simulink library "UDP_bus_create_lib"  (Simulink 7.2)
settings: Solver=ode45  StartTime=0.0  StopTime=10.0  RelTol=1e-3
libraries: simulink x1, UDP_lib x1
settings Model: Creator=cbuttril  LastModifiedBy=gtmdev

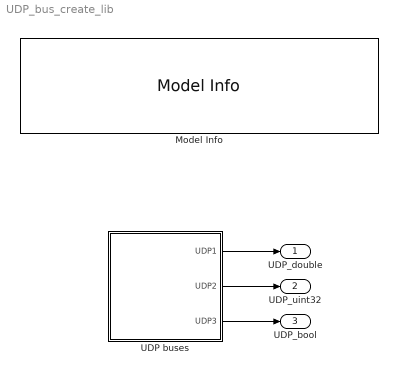
== system UDP_bus_create_lib ==
  Model Info : simulink/Model-Wide Utilities/Model Info  SystemSampleTime=-1  InitialBlockCM=None  BlockCM=None  Frame=on  DisplayStringWithTags=|  HorizontalTextAlignment=Center  LeftAlignmentValue=0.5  SourceBlockDiagram=UDP_bus_create_lib  TagMaxNumber=20
      | Developed using Matlab Release 2008b
      | 
      | SVN:%<ModelVersion>
      | Last modifed by %<LastModifiedBy> on %<LastModificationDate>
  UDP buses : Subsystem
  UDP_double : Outport  OutDataType=sfix(16)  OutScaling=2^0
  UDP_uint32 : Outport  Port=2  OutDataType=sfix(16)  OutScaling=2^0
  UDP_bool : Outport  Port=3  OutDataType=sfix(16)  OutScaling=2^0
  wires:
  UDP buses/1(UDP1) -> UDP_double/1
  UDP buses/2(UDP2) -> UDP_uint32/1
  UDP buses/3(UDP3) -> UDP_bool/1

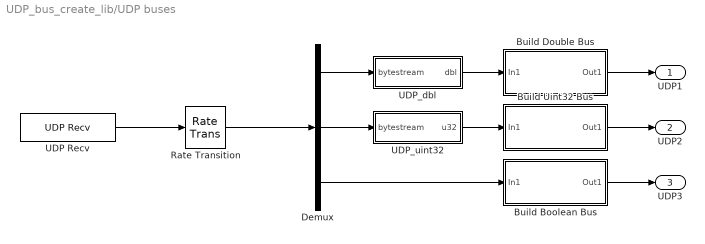
== system UDP_bus_create_lib/UDP buses ==
  Build Boolean Bus : Subsystem
  Build Double Bus : Subsystem
  Build Uint32 Bus : Subsystem
  Demux : Demux  Outputs=[1424,36,8]
  Rate Transition : RateTransition  OutPortSampleTime=Timestep
  UDP Recv : UDP_lib/UDP Recv  SystemSampleTime=-1  UDP_Port=5500  MSG_Length=1468
  UDP_dbl : Subsystem  mask(UDPPacker){IsBigEndian=0}
      mask prompts: IsBigEndian "Native Byte Ordering is Big Endian (boolean)"
      mask help: Takes a uint8 bytestream and remaps to vector of doubles, with byteswaping if required
  UDP_uint32 : Subsystem  mask(UDPPacker){IsBigEndian=0}
      mask prompts: IsBigEndian "Native Byte Ordering is Big Endian (boolean)"
      mask help: Takes a uint8 bytestream and remaps to vector of doubles, with byteswaping if required
  UDP1 : Outport  OutDataType=sfix(16)  OutScaling=2^0
  UDP2 : Outport  Port=2  OutDataType=sfix(16)  OutScaling=2^0
  UDP3 : Outport  Port=3  OutDataType=sfix(16)  OutScaling=2^0
  wires:
  UDP Recv/1 -> Rate Transition/1
  Demux/1 -> UDP_dbl/1(bytestream)
  Demux/2 -> UDP_uint32/1(bytestream)
  UDP_dbl/1(dbl) -> Build Double Bus/1(In1)
  UDP_uint32/1(u32) -> Build Uint32 Bus/1(In1)
  Demux/3 -> Build Boolean Bus/1(In1)
  Build Double Bus/1(Out1) -> UDP1/1
  Build Uint32 Bus/1(Out1) -> UDP2/1
  Build Boolean Bus/1(Out1) -> UDP3/1
  Rate Transition/1 -> Demux/1

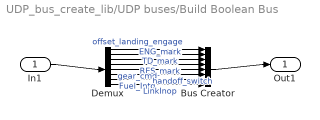
== system UDP_bus_create_lib/UDP buses/Build Boolean Bus ==
  In1 : Inport  OutDataType=sfix(16)  OutScaling=2^0
  Bus Creator : BusCreator  Inputs=8
  Demux : Demux  Outputs=8
  Out1 : Outport  OutDataType=sfix(16)  OutScaling=2^0
  wires:
  Demux/1 -> Bus Creator/1  "offset_landing_engage"
  Demux/2 -> Bus Creator/2  "TD_mark"
  Demux/3 -> Bus Creator/3  "ENG_mark"
  Demux/4 -> Bus Creator/4  "RES_mark"
  Demux/5 -> Bus Creator/5  "gear_cmd"
  Demux/6 -> Bus Creator/6  "handoff_switch"
  Demux/7 -> Bus Creator/7  "Fuel_Intg"
  Demux/8 -> Bus Creator/8  "LinkInop"
  In1/1 -> Demux/1
  Bus Creator/1 -> Out1/1

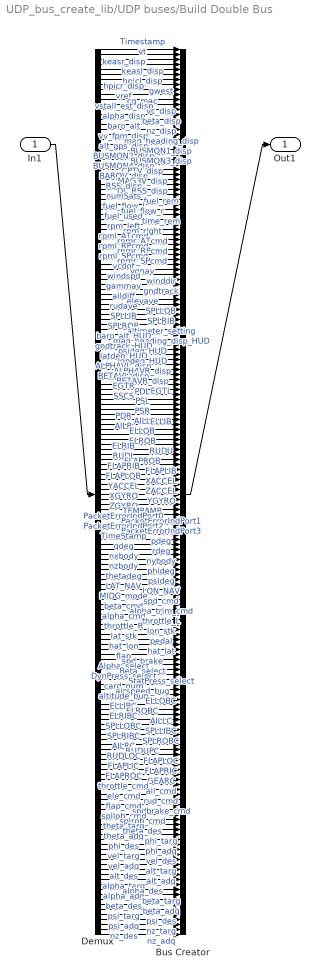
== system UDP_bus_create_lib/UDP buses/Build Double Bus ==
  In1 : Inport  OutDataType=sfix(16)  OutScaling=2^0
  Bus Creator : BusCreator  Inputs=178
  Demux : Demux  Outputs=178
  Out1 : Outport  OutDataType=sfix(16)  OutScaling=2^0
  wires:
  Demux/1 -> Bus Creator/1  "Timestamp"
  Demux/2 -> Bus Creator/2  "vc"
  Demux/3 -> Bus Creator/3  "vt"
  Demux/4 -> Bus Creator/4  "keasl_disp"
  Demux/5 -> Bus Creator/5  "keasr_disp"
  Demux/6 -> Bus Creator/6  "hpicl_disp"
  Demux/7 -> Bus Creator/7  "hpicr_disp"
  Demux/8 -> Bus Creator/8  "gwest"
  Demux/9 -> Bus Creator/9  "vref"
  Demux/10 -> Bus Creator/10  "cg_mac"
  Demux/11 -> Bus Creator/11  "vstall_est_disp"
  Demux/12 -> Bus Creator/12  "vc_disp"
  Demux/13 -> Bus Creator/13  "alpha_disp"
  Demux/14 -> Bus Creator/14  "beta_disp"
  Demux/15 -> Bus Creator/15  "baro_alt"
  Demux/16 -> Bus Creator/16  "nz_disp"
  Demux/17 -> Bus Creator/17  "vv_fpm_disp"
  Demux/18 -> Bus Creator/18  "mag_heading_disp"
  Demux/19 -> Bus Creator/19  "alt_gps_disp"
  Demux/20 -> Bus Creator/20  "BUSMON1_disp"
  Demux/21 -> Bus Creator/21  "BUSMON2_disp"
  Demux/22 -> Bus Creator/22  "BUSMON3_disp"
  Demux/23 -> Bus Creator/23  "BUSMON4_disp"
  Demux/24 -> Bus Creator/24  "CPTV_disp"
  Demux/25 -> Bus Creator/25  "BAROV_disp"
  Demux/26 -> Bus Creator/26  "MAG3V_disp"
  Demux/27 -> Bus Creator/27  "RSS_disp"
  Demux/28 -> Bus Creator/28  "DL_RSS_disp"
  Demux/29 -> Bus Creator/29  "numSats"
  Demux/30 -> Bus Creator/30  "fuel_rem"
  Demux/31 -> Bus Creator/31  "fuel_flow_l"
  Demux/32 -> Bus Creator/32  "fuel_flow_r"
  Demux/33 -> Bus Creator/33  "fuel_used"
  Demux/34 -> Bus Creator/34  "time_rem"
  Demux/35 -> Bus Creator/35  "rpm_left"
  Demux/36 -> Bus Creator/36  "rpm_right"
  Demux/37 -> Bus Creator/37  "rpml_ATcmd"
  Demux/38 -> Bus Creator/38  "rpmr_ATcmd"
  Demux/39 -> Bus Creator/39  "rpml_RPcmd"
  Demux/40 -> Bus Creator/40  "rpmr_RPcmd"
  Demux/41 -> Bus Creator/41  "rpml_SPcmd"
  Demux/42 -> Bus Creator/42  "rpmr_SPcmd"
  Demux/43 -> Bus Creator/43  "vcdot"
  Demux/44 -> Bus Creator/44  "vgnav"
  Demux/45 -> Bus Creator/45  "windspd"
  Demux/46 -> Bus Creator/46  "winddir"
  Demux/47 -> Bus Creator/47  "gammav"
  Demux/48 -> Bus Creator/48  "gndtrack"
  Demux/49 -> Bus Creator/49  "aildiff"
  Demux/50 -> Bus Creator/50  "elevave"
  Demux/51 -> Bus Creator/51  "rudave"
  Demux/52 -> Bus Creator/52  "SPLLOB"
  Demux/53 -> Bus Creator/53  "SPLLIB"
  Demux/54 -> Bus Creator/54  "SPLRIB"
  Demux/55 -> Bus Creator/55  "SPLROB"
  Demux/56 -> Bus Creator/56  "altimeter_setting"
  Demux/57 -> Bus Creator/57  "baro_alt_HUD"
  Demux/58 -> Bus Creator/58  "mag_heading_disp_HUD"
  Demux/59 -> Bus Creator/59  "gndtrack_HUD"
  Demux/60 -> Bus Creator/60  "psideg_HUD"
  Demux/61 -> Bus Creator/61  "latdeg_HUD"
  Demux/62 -> Bus Creator/62  "londeg_HUD"
  Demux/63 -> Bus Creator/63  "ALPHAVL_disp"
  Demux/64 -> Bus Creator/64  "ALPHAVR_disp"
  Demux/65 -> Bus Creator/65  "BETAVL_disp"
  Demux/66 -> Bus Creator/66  "BETAVR_disp"
  Demux/67 -> Bus Creator/67  "EGTR"
  Demux/68 -> Bus Creator/68  "EGTL"
  Demux/69 -> Bus Creator/69  "SSCS"
  Demux/70 -> Bus Creator/70  "PSL"
  Demux/71 -> Bus Creator/71  "PDL"
  Demux/72 -> Bus Creator/72  "PSR"
  Demux/73 -> Bus Creator/73  "PDR"
  Demux/74 -> Bus Creator/74  "AILL"
  Demux/75 -> Bus Creator/75  "AILR"
  Demux/76 -> Bus Creator/76  "ELLOB"
  Demux/77 -> Bus Creator/77  "ELLIB"
  Demux/78 -> Bus Creator/78  "ELROB"
  Demux/79 -> Bus Creator/79  "ELRIB"
  Demux/80 -> Bus Creator/80  "RUDU"
  Demux/81 -> Bus Creator/81  "RUDL"
  Demux/82 -> Bus Creator/82  "FLAPROB"
  Demux/83 -> Bus Creator/83  "FLAPRIB"
  Demux/84 -> Bus Creator/84  "FLAPLIB"
  Demux/85 -> Bus Creator/85  "FLAPLOB"
  Demux/86 -> Bus Creator/86  "XACCEL"
  Demux/87 -> Bus Creator/87  "YACCEL"
  Demux/88 -> Bus Creator/88  "ZACCEL"
  Demux/89 -> Bus Creator/89  "XGYRO"
  Demux/90 -> Bus Creator/90  "YGYRO"
  Demux/91 -> Bus Creator/91  "ZGYRO"
  Demux/92 -> Bus Creator/92  "TEMPAMB"
  Demux/93 -> Bus Creator/93  "PacketErrorIndPort0"
  Demux/94 -> Bus Creator/94  "PacketErrorIndPort1"
  Demux/95 -> Bus Creator/95  "PacketErrorIndPort2"
  Demux/96 -> Bus Creator/96  "PacketErrorIndPort3"
  Demux/97 -> Bus Creator/97  "TimeStamp"
  Demux/98 -> Bus Creator/98  "pdeg"
  Demux/99 -> Bus Creator/99  "qdeg"
  Demux/100 -> Bus Creator/100  "rdeg"
  Demux/101 -> Bus Creator/101  "nxbody"
  Demux/102 -> Bus Creator/102  "nybody"
  Demux/103 -> Bus Creator/103  "nzbody"
  Demux/104 -> Bus Creator/104  "phideg"
  Demux/105 -> Bus Creator/105  "thetadeg"
  Demux/106 -> Bus Creator/106  "psideg"
  Demux/107 -> Bus Creator/107  "LAT_NAV"
  Demux/108 -> Bus Creator/108  "LON_NAV"
  Demux/109 -> Bus Creator/109  "MIDG_mode"
  Demux/110 -> Bus Creator/110  "spd_cmd"
  Demux/111 -> Bus Creator/111  "beta_cmd"
  Demux/112 -> Bus Creator/112  "alpha_trim_cmd"
  Demux/113 -> Bus Creator/113  "alpha_cmd"
  Demux/114 -> Bus Creator/114  "throttle_L"
  Demux/115 -> Bus Creator/115  "throttle_R"
  Demux/116 -> Bus Creator/116  "lon_stk"
  Demux/117 -> Bus Creator/117  "lat_stk"
  Demux/118 -> Bus Creator/118  "pedal"
  Demux/119 -> Bus Creator/119  "hat_lon"
  Demux/120 -> Bus Creator/120  "hat_lat"
  Demux/121 -> Bus Creator/121  "flap"
  Demux/122 -> Bus Creator/122  "spd_brake"
  Demux/123 -> Bus Creator/123  "Alpha_select"
  Demux/124 -> Bus Creator/124  "Beta_select"
  Demux/125 -> Bus Creator/125  "DynPress_select"
  Demux/126 -> Bus Creator/126  "StatPress_select"
  Demux/127 -> Bus Creator/127  "card_num"
  Demux/128 -> Bus Creator/128  "airspeed_bug"
  Demux/129 -> Bus Creator/129  "altitude_bug"
  Demux/130 -> Bus Creator/130  "ELLOBC"
  Demux/131 -> Bus Creator/131  "ELLIBC"
  Demux/132 -> Bus Creator/132  "ELROBC"
  Demux/133 -> Bus Creator/133  "ELRIBC"
  Demux/134 -> Bus Creator/134  "AILLC"
  Demux/135 -> Bus Creator/135  "SPLLOBC"
  Demux/136 -> Bus Creator/136  "SPLLIBC"
  Demux/137 -> Bus Creator/137  "SPLRIBC"
  Demux/138 -> Bus Creator/138  "SPLROBC"
  Demux/139 -> Bus Creator/139  "AILRC"
  Demux/140 -> Bus Creator/140  "RUDUPC"
  Demux/141 -> Bus Creator/141  "RUDLOC"
  Demux/142 -> Bus Creator/142  "FLAPLOC"
  Demux/143 -> Bus Creator/143  "FLAPLIC"
  Demux/144 -> Bus Creator/144  "FLAPRIC"
  Demux/145 -> Bus Creator/145  "FLAPROC"
  Demux/146 -> Bus Creator/146  "GEARC"
  Demux/147 -> Bus Creator/147  "throttle_cmd"
  Demux/148 -> Bus Creator/148  "ail_cmd"
  Demux/149 -> Bus Creator/149  "ele_cmd"
  Demux/150 -> Bus Creator/150  "rud_cmd"
  Demux/151 -> Bus Creator/151  "flap_cmd"
  Demux/152 -> Bus Creator/152  "spdbrake_cmd"
  Demux/153 -> Bus Creator/153  "spllob_cmd"
  Demux/154 -> Bus Creator/154  "splrob_cmd"
  Demux/155 -> Bus Creator/155  "theta_targ"
  Demux/156 -> Bus Creator/156  "theta_des"
  Demux/157 -> Bus Creator/157  "theta_adq"
  Demux/158 -> Bus Creator/158  "phi_targ"
  Demux/159 -> Bus Creator/159  "phi_des"
  Demux/160 -> Bus Creator/160  "phi_adq"
  Demux/161 -> Bus Creator/161  "vel_targ"
  Demux/162 -> Bus Creator/162  "vel_des"
  Demux/163 -> Bus Creator/163  "vel_adq"
  Demux/164 -> Bus Creator/164  "alt_targ"
  Demux/165 -> Bus Creator/165  "alt_des"
  Demux/166 -> Bus Creator/166  "alt_adq"
  Demux/167 -> Bus Creator/167  "alpha_targ"
  Demux/168 -> Bus Creator/168  "alpha_des"
  Demux/169 -> Bus Creator/169  "alpha_adq"
  Demux/170 -> Bus Creator/170  "beta_targ"
  Demux/171 -> Bus Creator/171  "beta_des"
  Demux/172 -> Bus Creator/172  "beta_adq"
  Demux/173 -> Bus Creator/173  "psi_targ"
  Demux/174 -> Bus Creator/174  "psi_des"
  Demux/175 -> Bus Creator/175  "psi_adq"
  Demux/176 -> Bus Creator/176  "nz_targ"
  Demux/177 -> Bus Creator/177  "nz_des"
  Demux/178 -> Bus Creator/178  "nz_adq"
  In1/1 -> Demux/1
  Bus Creator/1 -> Out1/1

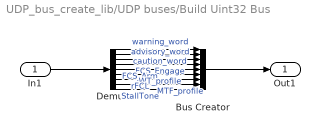
== system UDP_bus_create_lib/UDP buses/Build Uint32 Bus ==
  In1 : Inport  OutDataType=sfix(16)  OutScaling=2^0
  Bus Creator : BusCreator  Inputs=9
  Demux : Demux  Outputs=9
  Out1 : Outport  OutDataType=sfix(16)  OutScaling=2^0
  wires:
  Demux/1 -> Bus Creator/1  "warning_word"
  Demux/2 -> Bus Creator/2  "caution_word"
  Demux/3 -> Bus Creator/3  "advisory_word"
  Demux/4 -> Bus Creator/4  "FCS_Engage"
  Demux/5 -> Bus Creator/5  "FCS_Arm"
  Demux/6 -> Bus Creator/6  "WT_profile"
  Demux/7 -> Bus Creator/7  "rFCL"
  Demux/8 -> Bus Creator/8  "MTF_profile"
  Demux/9 -> Bus Creator/9  "StallTone"
  In1/1 -> Demux/1
  Bus Creator/1 -> Out1/1

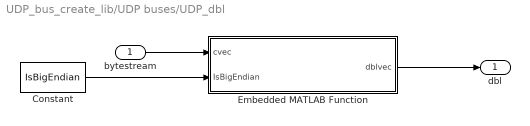
== system UDP_bus_create_lib/UDP buses/UDP_dbl ==
  bytestream : Inport  DataType=uint8  OutDataType=sfix(16)  OutScaling=2^0  OutDataTypeStr=uint8
  Constant : Constant  Value=IsBigEndian  OutDataTypeMode=boolean  OutDataType=sfix(16)  OutScaling=2^0  OutDataTypeStr=boolean
  Embedded MATLAB Function : Stateflow chart
  dbl : Outport  OutDataType=sfix(16)  OutScaling=2^0
  wires:
  bytestream/1 -> Embedded MATLAB Function/1(cvec)
  Embedded MATLAB Function/1(dblvec) -> dbl/1
  Constant/1 -> Embedded MATLAB Function/2(IsBigEndian)

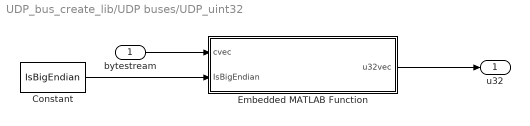
== system UDP_bus_create_lib/UDP buses/UDP_uint32 ==
  bytestream : Inport  DataType=uint8  OutDataType=sfix(16)  OutScaling=2^0  OutDataTypeStr=uint8
  Constant : Constant  Value=IsBigEndian  OutDataTypeMode=boolean  OutDataType=sfix(16)  OutScaling=2^0  OutDataTypeStr=boolean
  Embedded MATLAB Function : Stateflow chart
  u32 : Outport  DataType=uint32  OutDataType=sfix(16)  OutScaling=2^0  OutDataTypeStr=uint32
  wires:
  bytestream/1 -> Embedded MATLAB Function/1(cvec)
  Embedded MATLAB Function/1(u32vec) -> u32/1
  Constant/1 -> Embedded MATLAB Function/2(IsBigEndian)

== matlab function UDP buses/UDP_dbl/Embedded MATLAB Function ==
  data: cvec input uint8; IsBigEndian input boolean; dblvec output double
function dblvec = fcn(cvec,IsBigEndian)
Nv=length(cvec);
dblvec=zeros(Nv/8,1);
cmat=uint8(zeros(8,Nv/8));

% Note matlab swapbytes() function doesn't autocode, going manual
cmat=reshape(cvec,8,Nv/8);
if (~IsBigEndian)  % Little Endian, reorder
  cmat=flipud(cmat);
end
cvec=cmat(:);
dblvec=typecast(cvec,'double');

== matlab function UDP buses/UDP_uint32/Embedded MATLAB Function ==
  data: cvec input uint8; IsBigEndian input boolean; u32vec output uint32
function u32vec = fcn(cvec,IsBigEndian)
Nv=length(cvec);
u32vec=uint32(zeros(Nv/4,1));
cmat=uint8(zeros(4,Nv/4));

% Note matlab swapbytes() function doesn't autocode, going manual
cmat=reshape(cvec,4,Nv/4);
if (~IsBigEndian)  % Little Endian, reorder
  cmat=flipud(cmat);
end
cvec=cmat(:);
u32vec=typecast(cvec,'uint32');
